simulink model "adaptive_mit_rule"  (R2015b)
settings: Solver=VariableStepAuto  StartTime=0.0  StopTime=100  RelTol=1e-3
settings Model: Creator=Laxus  LastModifiedBy=uchiha

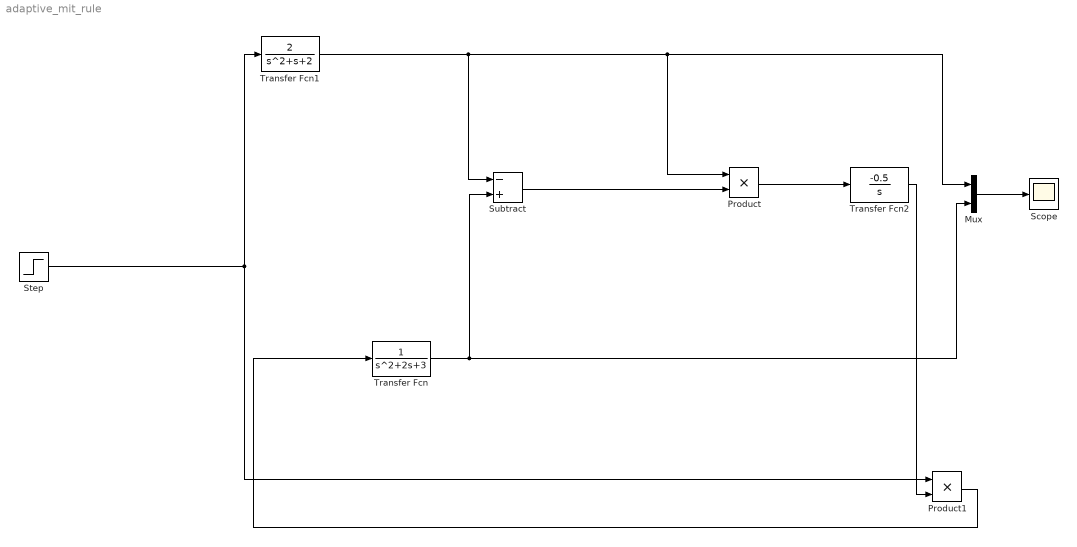
== system adaptive_mit_rule ==
  Mux : Mux  Inputs=2
  Product : Product
  Product1 : Product
  Scope : Scope
  Step : Step  After=2.5  SampleTime=0
  Subtract : Sum  Inputs=-+
  Transfer Fcn : TransferFcn  Denominator=[1 2 3]
  Transfer Fcn1 : TransferFcn  Numerator=[2]  Denominator=[1 1 2]  ContinuousStateAttributes='reference'
  Transfer Fcn2 : TransferFcn  Numerator=[-0.5]  Denominator=[1 0]
  wires:
  Transfer Fcn1/1 -> Subtract/1, Product/1, Mux/1
  Subtract/1 -> Product/2
  Product/1 -> Transfer Fcn2/1
  Transfer Fcn2/1 -> Product1/2
  Product1/1 -> Transfer Fcn/1
  Mux/1 -> Scope/1
  Step/1 -> Transfer Fcn1/1, Product1/1
  Transfer Fcn/1 -> Subtract/2, Mux/2
